simulink model "AC_motor_ao"  (R2019a)
settings: Solver=VariableStepAuto  StartTime=0.0  StopTime=0.16  RelTol=1e-3
values from neighbouring files (symbols this model uses):
  J = 0.0011    [Tham_So_AC_motor_ao.m]
  Lr = 0.7015    [Tham_So_AC_motor_ao.m]
  Ls = 0.663    [Tham_So_AC_motor_ao.m]
  M = 0.624    [Tham_So_AC_motor_ao.m]
  p = 2    [Dac_tinhCo_dong_co_KD_roto_longSoc.m]    (also in Tham_So_AC_motor_ao.m)
  Rr = 15.08    [Tham_So_AC_motor_ao.m]
  Rs = 16.39    [Tham_So_AC_motor_ao.m]
libraries: powerlib x1
settings Model: Creator=Admin  LastModifiedBy=Admin

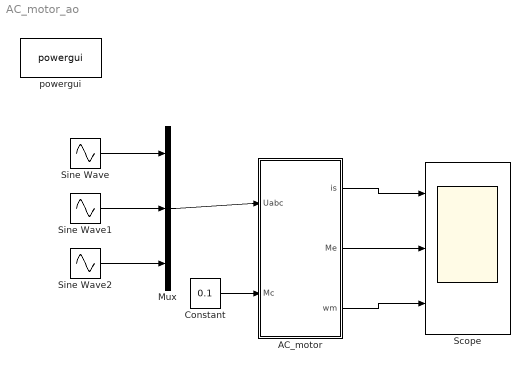
== system AC_motor_ao ==
  AC_motor : Subsystem
  Constant : Constant  Value=0.1
  Mux : Mux  Inputs=3
  Scope : Scope  NumInputPorts=3
  Sine Wave : Sin  Amplitude=220  Frequency=2*pi*50  SampleTime=0
  Sine Wave1 : Sin  Amplitude=220  Frequency=2*pi*50  Phase=-2*pi/3  SampleTime=0
  Sine Wave2 : Sin  Amplitude=220  Frequency=2*pi*50  Phase=2*pi/3  SampleTime=0
  powergui : powerlib/powergui  Priority=1  SimulationMode=Continuous  SampleTime=50e-6  frequency=60  Iterations=50  frequencyindice=60  Pbase=100e6  ErrMax=1e-4  UnitsV=kV  UnitsW=MW  buscounter=0  FunctionMessages=off  echomessages=off  EnableUseOfTLC=off  CurrentSourceSwitches=off  DisableSnubberDevices=off  DisableRonSwitches=off  DisableVfSwitches=off  DisplayEquations=off  AutomaticDiscreteSolvers=off  SolverType=Tustin/Backward Euler (TBE)  Interpol=off  ExternalGateDelay=off  methode=off  Ts=100  x0status=blocks  SPID=on  SwTol=0  HookPort=off  NonlinearTolerance=0  nMaxIteration=15  ContinueOnMaxIteration=off  RestoreLinks=warning  ResistiveCurrentMeasurement=off  Frange=[0:2:500]  Ylog=off  Xlog=on  ShowGrid=off  save=off  variable=ZData  structure=0  ZoomFFT=off  StartTime=0.0  cycles=1  DisplayStyle=1  fundamental=60  FreqAxis=off  MaxFrequency=1000  frequencyindicesteady=1  RmsSteady=1  display=off
      settings: SourceProductName=Simscape Electrical
  wires:
  Sine Wave/1 -> Mux/1
  Mux/1 -> AC_motor/1(Uabc)
  Constant/1 -> AC_motor/2(Mc)
  AC_motor/1(is) -> Scope/1
  AC_motor/2(Me) -> Scope/2
  AC_motor/3(wm) -> Scope/3
  Sine Wave1/1 -> Mux/2
  Sine Wave2/1 -> Mux/3

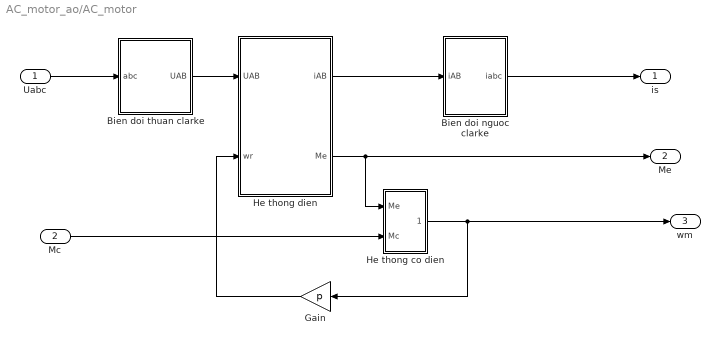
== system AC_motor_ao/AC_motor ==
  Uabc : Inport
  Mc : Inport  Port=2
  Bien doi nguoc clarke : Subsystem
  Bien doi thuan clarke : Subsystem
  Gain : Gain  Gain=p
  He thong co dien : Subsystem
  "He thong dien " : Subsystem
  is : Outport
  Me : Outport  Port=2
  wm : Outport  Port=3
  wires:
  Mc/1 -> He thong co dien/2(Mc)
  Uabc/1 -> Bien doi thuan clarke/1(abc)
  Gain/1 -> "He thong dien "/2(wr)
  "He thong dien "/1(iAB) -> Bien doi nguoc clarke/1(iAB)
  Bien doi thuan clarke/1(UAB) -> "He thong dien "/1(UAB)
  He thong co dien/1(wm) -> wm/1, Gain/1
  "He thong dien "/2(Me) -> Me/1, He thong co dien/1(Me)
  Bien doi nguoc clarke/1(iabc) -> is/1

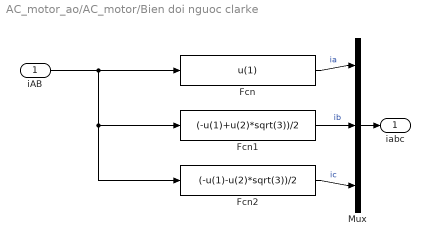
== system AC_motor_ao/AC_motor/Bien doi nguoc clarke ==
  iAB : Inport
  Fcn : Fcn  Expr=u(1)
  Fcn1 : Fcn  Expr=(-u(1)+u(2)*sqrt(3))/2
  Fcn2 : Fcn  Expr=(-u(1)-u(2)*sqrt(3))/2
  Mux : Mux  Inputs=3
  iabc : Outport
  wires:
  Fcn/1 -> Mux/1  "ia"
  iAB/1 -> Fcn1/1, Fcn2/1, Fcn/1
  Fcn1/1 -> Mux/2  "ib"
  Fcn2/1 -> Mux/3  "ic"
  Mux/1 -> iabc/1

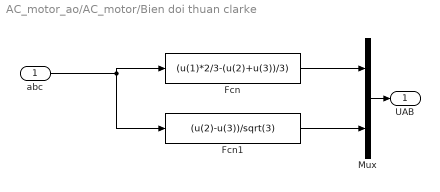
== system AC_motor_ao/AC_motor/Bien doi thuan clarke ==
  abc : Inport
  Fcn : Fcn  Expr=(u(1)*2/3-(u(2)+u(3))/3)
  Fcn1 : Fcn  Expr=(u(2)-u(3))/sqrt(3)
  Mux : Mux  Inputs=2
  UAB : Outport
  wires:
  Mux/1 -> UAB/1
  Fcn/1 -> Mux/1
  Fcn1/1 -> Mux/2
  abc/1 -> Fcn/1, Fcn1/1

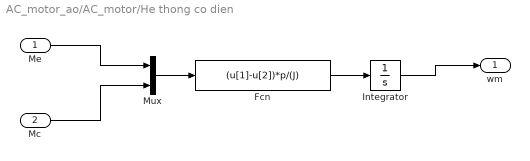
== system AC_motor_ao/AC_motor/He thong co dien ==
  Me : Inport
  Mc : Inport  Port=2
  Fcn : Fcn  Expr=(u[1]-u[2])*p/(J)
  Integrator : Integrator
  Mux : Mux  Inputs=2
  wm : Outport
  wires:
  Fcn/1 -> Integrator/1
  Mc/1 -> Mux/2
  Me/1 -> Mux/1
  Mux/1 -> Fcn/1
  Integrator/1 -> wm/1

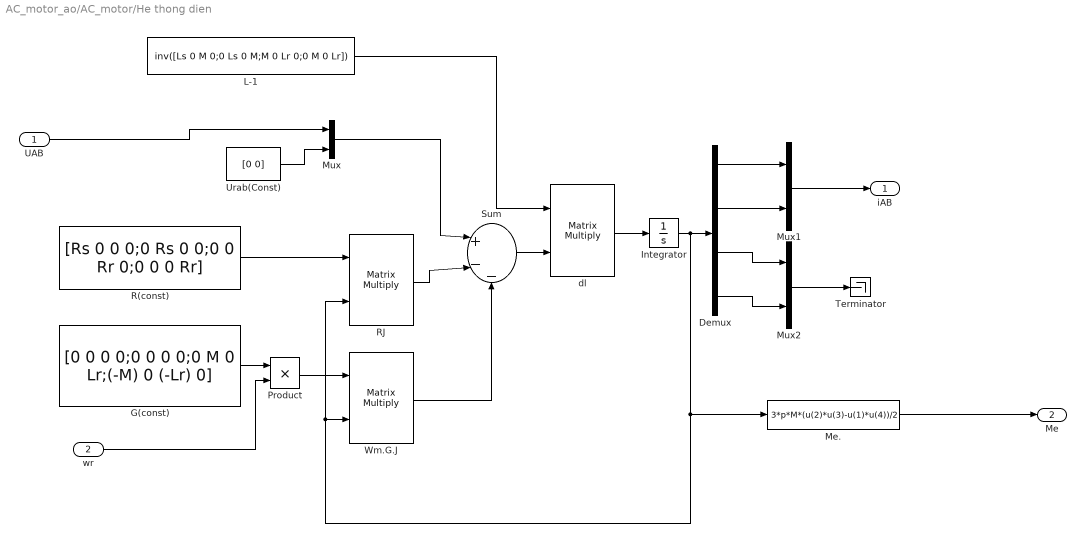
== system AC_motor_ao/AC_motor/He thong dien  ==
  UAB : Inport
  wr : Inport  Port=2
  Demux : Demux
  G(const) : Constant  Value=[0 0 0 0;0 0 0 0;0 M 0 Lr;(-M) 0 (-Lr) 0]
  Integrator : Integrator
  L-1 : Constant  Value=inv([Ls 0 M 0;0 Ls 0 M;M 0 Lr 0;0 M 0 Lr])
  Me. : Fcn  Expr=3*p*M*(u(2)*u(3)-u(1)*u(4))/2
  Mux : Mux  Inputs=2
  Mux1 : Mux  Inputs=2
  Mux2 : Mux  Inputs=2
  Product : Product
  R(const) : Constant  Value=[Rs 0 0 0;0 Rs 0 0;0 0 Rr 0;0 0 0 Rr]
  RJ : Product  Multiplication=Matrix(*)
  Sum : Sum  Inputs=|+--
  Terminator : Terminator
  Urab(Const) : Constant  Value=[0 0]
  Wm.G.J : Product  Multiplication=Matrix(*)
  dl : Product  Multiplication=Matrix(*)
  iAB : Outport
  Me : Outport  Port=2
  wires:
  Demux/3 -> Mux2/1
  R(const)/1 -> RJ/1
  G(const)/1 -> Product/1
  Integrator/1 -> Wm.G.J/2, RJ/2, Me./1, Demux/1
  Urab(Const)/1 -> Mux/2
  Demux/2 -> Mux1/2
  Product/1 -> Wm.G.J/1
  Mux/1 -> Sum/1
  Demux/1 -> Mux1/1
  Demux/4 -> Mux2/2
  L-1/1 -> dl/1
  RJ/1 -> Sum/2
  Sum/1 -> dl/2
  Mux1/1 -> iAB/1
  dl/1 -> Integrator/1
  UAB/1 -> Mux/1
  wr/1 -> Product/2
  Me./1 -> Me/1
  Mux2/1 -> Terminator/1
  Wm.G.J/1 -> Sum/3
